simulink model "Simple_Model_Packaging_power_estimate"  (R2022b)
settings: Solver=VariableStepAuto  StartTime=0.0  StopTime=0.001  RelTol=1e-3
InitFcn:
  | Parameter_Initialize_1
undefined symbols (not defined in the file or in its folder): gcbh, magnitude, model, rcfiltgaincompat, rsgenpoly
libraries: simulink x5, commsynccomp2 x3, commblkcod2 x2, commfilt2 x2, commdigbbndam3 x2, commrandsrc3 x2, commseqgen3 x2, commsink2 x1, commdigbbndfm2 x1, commchan3 x1, dspsigops x1, commdigbbndcpm2 x1
settings Model: Creator=89778  LastModifiedBy=89778

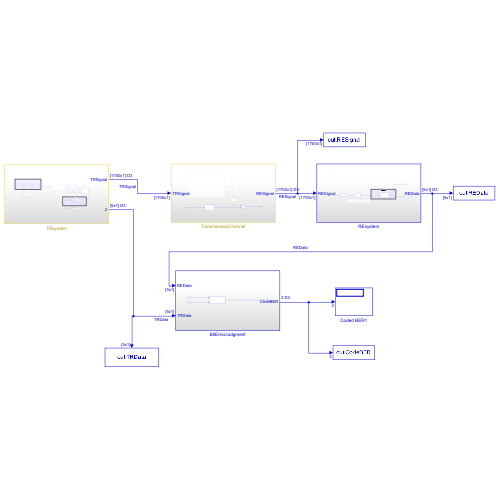
[thumbnail: Simulink's stored preview of the top-level diagram]
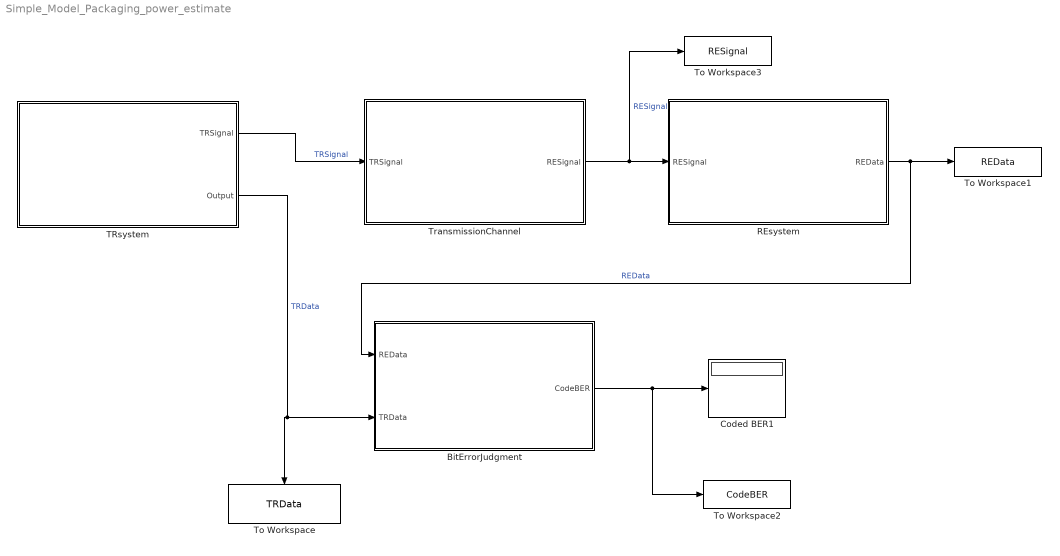
== system Simple_Model_Packaging_power_estimate ==
  BitErrorJudgment : Subsystem
  Coded BER1 : Display
  REsystem : Subsystem
  TRsystem : Subsystem
  To Workspace : ToWorkspace  VariableName=TRData  SaveFormat=Timeseries  SampleTime=-1
  To Workspace1 : ToWorkspace  VariableName=REData  SaveFormat=Timeseries  SampleTime=-1
  To Workspace2 : ToWorkspace  VariableName=CodeBER  SaveFormat=Timeseries  SampleTime=-1
  To Workspace3 : ToWorkspace  VariableName=RESignal  SaveFormat=Timeseries  SampleTime=-1
  TransmissionChannel : Subsystem
  wires:
  REsystem/1(REData) -> BitErrorJudgment/1(REData), To Workspace1/1  "REData"
  TransmissionChannel/1(RESignal) -> To Workspace3/1, REsystem/1(RESignal)  "RESignal"
  TRsystem/1(TRSignal) -> TransmissionChannel/1(TRSignal)  "TRSignal"
  TRsystem/2(Output) -> BitErrorJudgment/2(TRData), To Workspace/1  "TRData"
  BitErrorJudgment/1(CodeBER) -> To Workspace2/1, Coded BER1/1

== system Simple_Model_Packaging_power_estimate/BitErrorJudgment ==
  REData : Inport
  TRData : Inport  Port=2
  Bit Error Rate Calculation : Subsystem
      mask Display:
      | disp('Bit Error\nRate\nCalculation')
      | port_label('input', 1, 'Tx')
      | port_label('input', 2, 'Rx')
  CodeBER : Outport
  wires:
  TRData/1 -> Bit Error Rate Calculation/1(In1)
  REData/1 -> Bit Error Rate Calculation/2(In2)
  Bit Error Rate Calculation/1(Out1) -> CodeBER/1  "CodeBER"

== system Simple_Model_Packaging_power_estimate/REsystem ==
  note: 接收端解码
  note: 注意此处的延时设置，使得RS解码对齐信源部分，并在后续的码元比较时舍弃前三个编码周期(帧周期)的比特位
  RESignal : Inport
  Delay : Delay  DelayLength=model.Parameters.RE.Delay.Sample_length  InitialCondition=0  InputProcessing=Columns as channels (frame based)
  Integer-Output RS Decoder1 : commblkcod2/Integer-Output RS Decoder  n=model.Parameters.RE.Integer_Output_RS_Decoder1.Codeword_Length  k=model.Parameters.RE.Integer_Output_RS_Decoder1.Message_Length  specShortening=off  shortenedK=3  specGenPoly=off  genPoly=rsgenpoly(7, 3, [], [], 'double')  specPrimPoly=off  prPoly='X^3 + X + 1'  specPuncture=off  punctVec=[ones(2,1); zeros(2,1)]  specErasurePort=off  showNumErr=on
  Raised Cosine Receive Filter : commfilt2/Raised Cosine Receive Filter  filtType=Square root  R=model.Parameters.RE.Raised_Cosine_Receive_Filter.Rolloff_factor  filtSpan=model.Parameters.RE.Raised_Cosine_Receive_Filter.Filter_span_in_symbols  N=model.Parameters.RE.Raised_Cosine_Receive_Filter.Input_samples_per_symbol  downFactor=model.Parameters.RE.Raised_Cosine_Receive_Filter.Decimation_factor  downOffset=0  filterGain=rcfiltgaincompat(gcbh)  InputProcessing=Columns as channels (frame based)  RateOptions=Enforce single-rate processing  framing=Mute  checkCoeff=off  variableName=rcRxFilt  currentFiltSpan=10  D=5  inputOffset=0  sampMode=Mute  saveAsFlag=0  rateMode=Downsampling  checkGain=Normalized  launchFVT=on  roundingMode=Floor  overflowMode=off  coeffDataTypeStr=Inherit: Same word length as input  coeffMin=[]  coeffMax=[]  coeffLastDataTypeStr=Inherit: Same word length as input  accumDataTypeStr=Inherit: Same as product output  accumLastDataTypeStr=Inherit: Same as product output  outputDataTypeStr=Inherit: Same as accumulator  outputMin=[]  outputMax=[]  outputLastDataTypeStr=Inherit: Same as accumulator
  Rectangular QAM Demodulator Baseband : commdigbbndam3/Rectangular QAM Demodulator Baseband  M=model.Parameters.RE.Rectangular_QAM_Demodulator_Baseband.M_Number  OutType=Integer  DecType=Hard decision  VarSource=Dialog  Variance=1  Dec=Gray  Mapping=[0:15]  PowType=Min. distance between symbols  MinDist=model.Parameters.RE.Rectangular_QAM_Demodulator_Baseband.Minimum_distance  AvgPow=1  PeakPow=1  Ph=0  outDtype1=Inherit via internal rule  outDtype2=Inherit via internal rule  derotateFactorWordLen=16  derotateFactorDataTypeStr=Inherit: Same word length as input  derotateFactorLastDataTypeStr=Inherit: Same word length as input  denormFactorWordLen=16  denormFactorDataTypeStr=Inherit: Same word length as input  denormFactorLastDataTypeStr=Inherit: Same word length as input  prodOutWordLen=32  prodOutOverflowMode=Wrap  prodOutRoundingMode=Floor  prodOutOvFlMode=off  prodOutOvFlModeLastStrValue=off  sumWordLen=32
  Total Number of Corrected Errors : Display
  REData : Outport
  wires:
  Integer-Output RS Decoder1/2 -> Total Number of Corrected Errors/1
  Rectangular QAM Demodulator Baseband/1 -> Delay/1
  Delay/1 -> Integer-Output RS Decoder1/1
  Raised Cosine Receive Filter/1 -> Rectangular QAM Demodulator Baseband/1
  RESignal/1 -> Raised Cosine Receive Filter/1  "RESignal"
  Integer-Output RS Decoder1/1 -> REData/1  "REData"

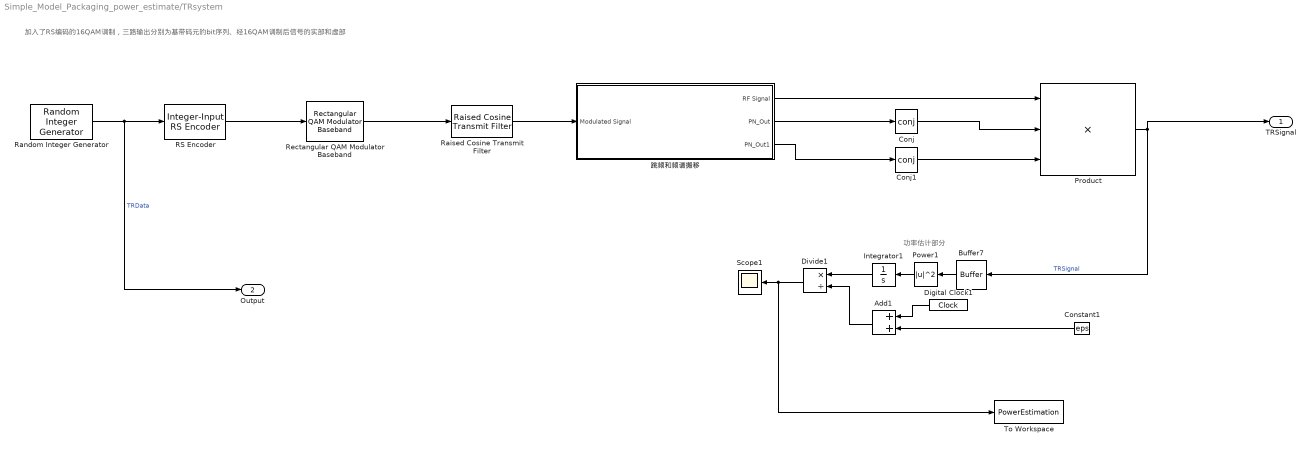
== system Simple_Model_Packaging_power_estimate/TRsystem ==
  note: 功率估计部分
  note: 加入了RS编码的16QAM调制，三路输出分别为基带码元的bit序列、经16QAM调制后信号的实部和虚部
  Add1 : Sum
  Buffer7 : Buffer  N=1  OutputFrames=off
  Conj : Math  Operator=conj
  Conj1 : Math  Operator=conj
  Constant1 : Constant  Value=eps  SampleTime=model.Parameters.TR.system_frame_speed
  Digital Clock1 : DigitalClock  SampleTime=model.Parameters.TR.system_frame_speed
  Divide1 : Product  Inputs=*/
  Integrator1 : Integrator
  Power1 : Math  Operator=magnitude^2
  Product : Product  Inputs=3
  RS Encoder : commblkcod2/Integer-Input RS Encoder  n=model.Parameters.TR.RS_Encoder.Codeword_Length  k=model.Parameters.TR.RS_Encoder.Message_Length  specShortening=off  shortenedK=3  specGenPoly=off  genPoly=rsgenpoly(7,3)  specPrimPoly=off  prPoly=[1 0 1 1]  specPuncture=off  punctVec=[ones(2,1); zeros(2,1)]
  Raised Cosine Transmit Filter : commfilt2/Raised Cosine Transmit Filter  filtType=Square root  R=model.Parameters.TR.Raised_Cosine_Transmit_Filter.Rolloff_factor  filtSpan=model.Parameters.TR.Raised_Cosine_Transmit_Filter.Filter_span_in_symbols  N=model.Parameters.TR.Raised_Cosine_Transmit_Filter.Output_samples_per_symbol  filterGain=rcfiltgaincompat(gcbh)  InputProcessing=Columns as channels (frame based)  RateOptions=Enforce single-rate processing  framing=Mute  checkCoeff=off  variableName=rcTxFilt  checkGain=Normalized  sampMode=Mute  saveAsFlag=0  currentFiltSpan=10  D=(10)/2  launchFVT=on  roundingMode=Floor  overflowMode=off  coeffDataTypeStr=Inherit: Same word length as input  coeffMin=[]  coeffMax=[]  coeffLastDataTypeStr=Inherit: Same word length as input  outputDataTypeStr=Inherit: Same as accumulator  outputMin=[]  outputMax=[]  outputLastDataTypeStr=Inherit: Same as accumulator
  Random Integer Generator : commrandsrc3/Random Integer Generator  SetSize=model.Parameters.TR.Random_Integer_Generator.SetSize  SeedSource=Auto  Seed=4  SampleTime=model.Parameters.TR.Random_Integer_Generator.Random_Sample_Time  SamplesPerFrame=model.Parameters.TR.Random_Integer_Generator.Samples_per_frame  OutputDataType=double  SimulateUsing=Interpreted execution
  Rectangular QAM Modulator Baseband : commdigbbndam3/Rectangular QAM Modulator Baseband  M=model.Parameters.TR.Rectangular_QAM_Modulator_Baseband.M_Number  InType=Integer  Enc=Gray  Mapping=[0:15]  PowType=Min. distance between symbols  MinDist=model.Parameters.TR.Rectangular_QAM_Modulator_Baseband.Minimum_distance  AvgPow=1  PeakPow=1  Ph=0  outDtype=double  outWordLen=16  outUDDataType=sfix(16)  outFracLenMode=Best precision  outFracLen=15  outDataTypeStr=double  outLastDataTypeStr=double
      settings: LibrarySourceBlock=|
      | commhdldigbbndam/Rectangular QAM
      | Modulator
      | Baseband
  Scope1 : Scope
  To Workspace : ToWorkspace  VariableName=PowerEstimation  SaveFormat=Timeseries  SampleTime=-1
  跳频和频谱搬移 : Subsystem
  TRSignal : Outport
  Output : Outport  Port=2
  wires:
  RS Encoder/1 -> Rectangular QAM Modulator Baseband/1
  跳频和频谱搬移/1(RF Signal) -> Product/1
  Random Integer Generator/1 -> Output/1, RS Encoder/1  "TRData"
  跳频和频谱搬移/3(PN_Out1) -> Conj1/1
  跳频和频谱搬移/2(PN_Out) -> Conj/1
  Raised Cosine Transmit Filter/1 -> 跳频和频谱搬移/1(Modulated Signal)
  Add1/1 -> Divide1/2
  Digital Clock1/1 -> Add1/1
  Divide1/1 -> To Workspace/1, Scope1/1
  Conj/1 -> Product/2
  Integrator1/1 -> Divide1/1
  Conj1/1 -> Product/3
  Constant1/1 -> Add1/2
  Rectangular QAM Modulator Baseband/1 -> Raised Cosine Transmit Filter/1
  Product/1 -> TRSignal/1, Buffer7/1  "TRSignal"
  Buffer7/1 -> Power1/1
  Power1/1 -> Integrator1/1

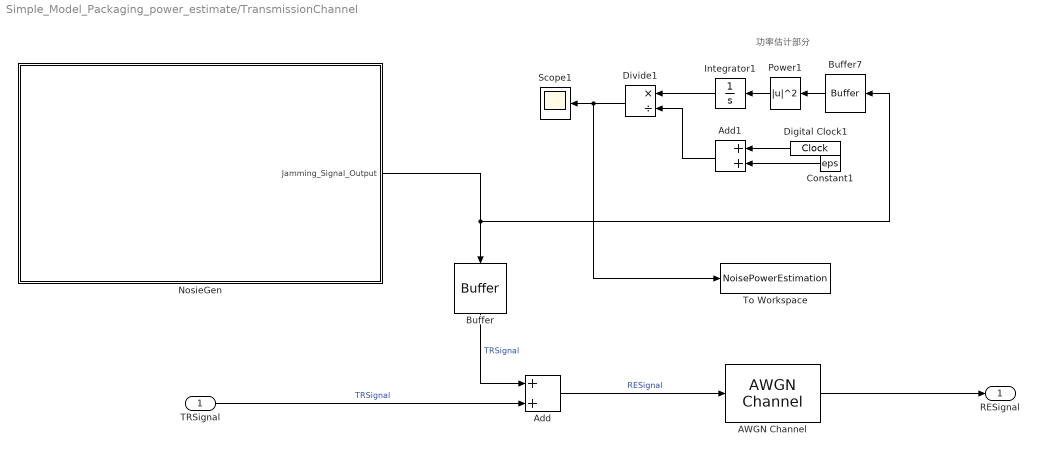
== system Simple_Model_Packaging_power_estimate/TransmissionChannel ==
  note: 功率估计部分
  TRSignal : Inport
  AWGN Channel : commchan3/AWGN Channel  InputProcessing=Columns as channels (frame based)  seed=67  noiseMode="Signal to noise ratio  (SNR)"  EbNodB=10  EsNodB=10  SNRdB=model.Parameters.Channel.Awgn.SNR  bitsPerSym=1  Ps=model.Parameters.Channel.Awgn.input_power  Tsym=1  variance=1
  Add : Sum
  Add1 : Sum
  Buffer : Buffer  N=model.Parameters.TR.rolloff_later_data_length  OutputFrames=off
  Buffer7 : Buffer  N=1  OutputFrames=off
  Constant1 : Constant  Value=eps  SampleTime=model.Parameters.TR.system_frame_speed
  Digital Clock1 : DigitalClock  SampleTime=model.Parameters.NoiseGen.NoiseTs
  Divide1 : Product  Inputs=*/
  Integrator1 : Integrator
  NosieGen : Subsystem
  Power1 : Math  Operator=magnitude^2
  Scope1 : Scope
  To Workspace : ToWorkspace  VariableName=NoisePowerEstimation  SaveFormat=Timeseries  SampleTime=-1
  RESignal : Outport
  wires:
  Add/1 -> AWGN Channel/1  "RESignal"
  NosieGen/1(Jamming_Signal_Output) -> Buffer7/1, Buffer/1
  AWGN Channel/1 -> RESignal/1
  TRSignal/1 -> Add/2  "TRSignal"
  Buffer/1 -> Add/1  "TRSignal"
  Power1/1 -> Integrator1/1
  Add1/1 -> Divide1/2
  Buffer7/1 -> Power1/1
  Divide1/1 -> To Workspace/1, Scope1/1
  Constant1/1 -> Add1/2
  Integrator1/1 -> Divide1/1
  Digital Clock1/1 -> Add1/1

== system Simple_Model_Packaging_power_estimate/BitErrorJudgment/Bit Error Rate Calculation ==
  In1 : Inport
  In2 : Inport  Port=2
  Error Rate Calculation : commsink2/Error Rate Calculation  N=model.Parameters.BER.Error_Rate_Calculation.receive_Delay  st_delay=0  cp_mode=Entire frame  subframe=[]  PMode=Port  WsName=ErrorVec  RsMode2=off  stop=on  numErr=100  maxBits=1e9
  Integer to Bit Converter : simulink/Logic and Bit Operations/Integer to Bit Converter  nbits=model.Parameters.BER.Integer_to_Bit_Converter.M  signedInputValues=Unsigned  bitOrder=MSB first  outDtype=Inherit via internal rule
      settings: LibrarySourceBlock=|
      | commutil2/Integer to Bit
      | Converter
  Integer to Bit Converter1 : simulink/Logic and Bit Operations/Integer to Bit Converter  nbits=model.Parameters.BER.Integer_to_Bit_Converter1.M  signedInputValues=Unsigned  bitOrder=MSB first  outDtype=Inherit via internal rule
      settings: LibrarySourceBlock=|
      | commutil2/Integer to Bit
      | Converter
  Out1 : Outport  VectorParamsAs1DForOutWhenUnconnected=off
  wires:
  Integer to Bit Converter/1 -> Error Rate Calculation/1
  Integer to Bit Converter1/1 -> Error Rate Calculation/2
  In1/1 -> Integer to Bit Converter/1
  Error Rate Calculation/1 -> Out1/1
  In2/1 -> Integer to Bit Converter1/1

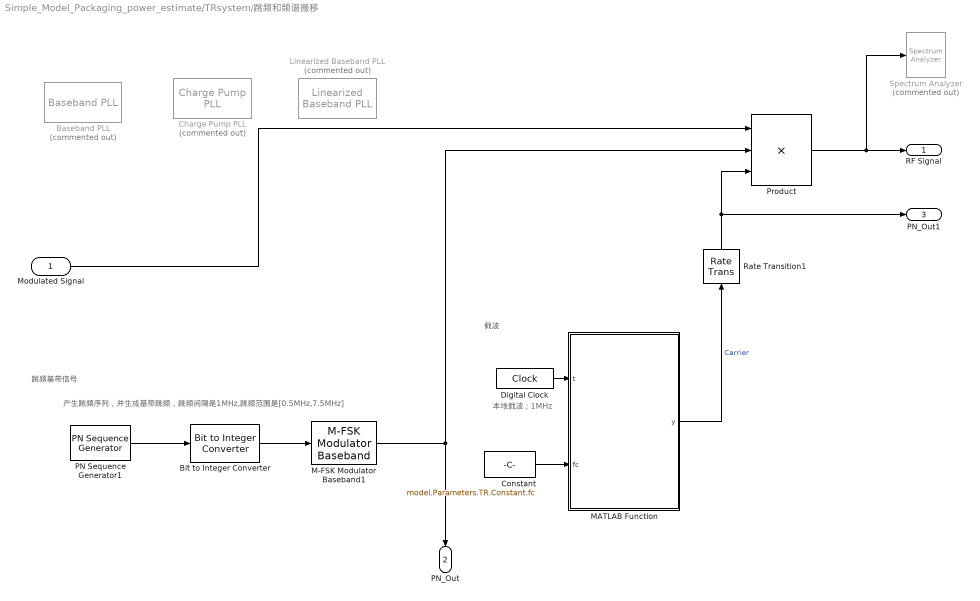
== system Simple_Model_Packaging_power_estimate/TRsystem/跳频和频谱搬移 ==
  note: 本地载波 ; 1MHz
  note: 产生跳频序列，并生成基带跳频，跳频间隔是1MHz,跳频范围是[0.5MHz,7.5MHz]
  note: 跳频基带信号
  note: 载波
  Modulated Signal : Inport
  Baseband PLL : commsynccomp2/Baseband PLL  Commented=on  Fn="[3.0002  0  40002]"  Fd="[1   67.46   2270.9   40002]"  Kvco=1
  Bit to Integer Converter : simulink/Logic and Bit Operations/Bit to Integer Converter  nbits=model.Parameters.TR.Bit_to_Integer_Converter.M  bitOrder=MSB first  signedOutputValues=Unsigned  outDtype=double  outDtypeSigned=Inherit via internal rule
  Charge Pump PLL : commsynccomp2/Charge Pump PLL  Commented=on  Fn="[3.0002  0  40002]"  Fd="[1   67.46   2270.9   40002]"  Kvco=1  Fc=100  Ph=0  Ac=1
  Constant : Constant  Value=model.Parameters.TR.Constant.fc
  Digital Clock : DigitalClock  SampleTime=model.Parameters.TR.Digital_Clock.fc_Ts
  Linearized Baseband PLL : commsynccomp2/Linearized Baseband PLL  Commented=on  Fn="[3.0002  0  40002]"  Fd="[1   67.46   2270.9   40002]"  Kvco=1
  M-FSK Modulator Baseband1 : commdigbbndfm2/M-FSK Modulator Baseband  M=model.Parameters.TR.M_FSK_Modulator_Baseband1.M_ary_number  InType=Integer  Enc=Gray  freqSep=model.Parameters.TR.M_FSK_Modulator_Baseband1.Frequency_separation  phaseType=Continuous  numSamp=model.Parameters.TR.M_FSK_Modulator_Baseband1.Samples_per_symbol  RateOptions=Enforce single-rate processing  outDataType=double
  MATLAB Function : MATLAB Function  TreatAsAtomicUnit=on
  PN Sequence Generator1 : commseqgen3/PN Sequence Generator  poly=model.Parameters.TR.PN_Sequence_Generator1.Generator_polynomial  ini_sta=model.Parameters.TR.PN_Sequence_Generator1.Initial_states  outBitMaskSource=Dialog parameter  shift=0  outVarSiz=off  maxOutSizeMode=Dialog parameter  maxOutSize=[10 1]  Ts=model.Parameters.TR.PN_Sequence_Generator1.Sample_time  sampPerFrame=model.Parameters.TR.PN_Sequence_Generator1.Samples_per_frame  reset=off  bitPackedOutputs=off  outDataType=double  numPackedBits=5  bitPackDataSigned=off  bitPackedOutDType=double
  Product : Product  Inputs=3
  Rate Transition1 : RateTransition
  Spectrum Analyzer : SpectrumAnalyzer  Commented=on
  RF Signal : Outport
  PN_Out : Outport  Port=2
  PN_Out1 : Outport  Port=3
  wires:
  Bit to Integer Converter/1 -> M-FSK Modulator Baseband1/1
  PN Sequence Generator1/1 -> Bit to Integer Converter/1
  Modulated Signal/1 -> Product/1
  Product/1 -> Spectrum Analyzer/1, RF Signal/1
  Digital Clock/1 -> MATLAB Function/1(t)
  M-FSK Modulator Baseband1/1 -> Product/2, PN_Out/1
  MATLAB Function/1(y) -> Rate Transition1/1  "Carrier"
  Rate Transition1/1 -> Product/3, PN_Out1/1
  Constant/1 -> MATLAB Function/2(fc)

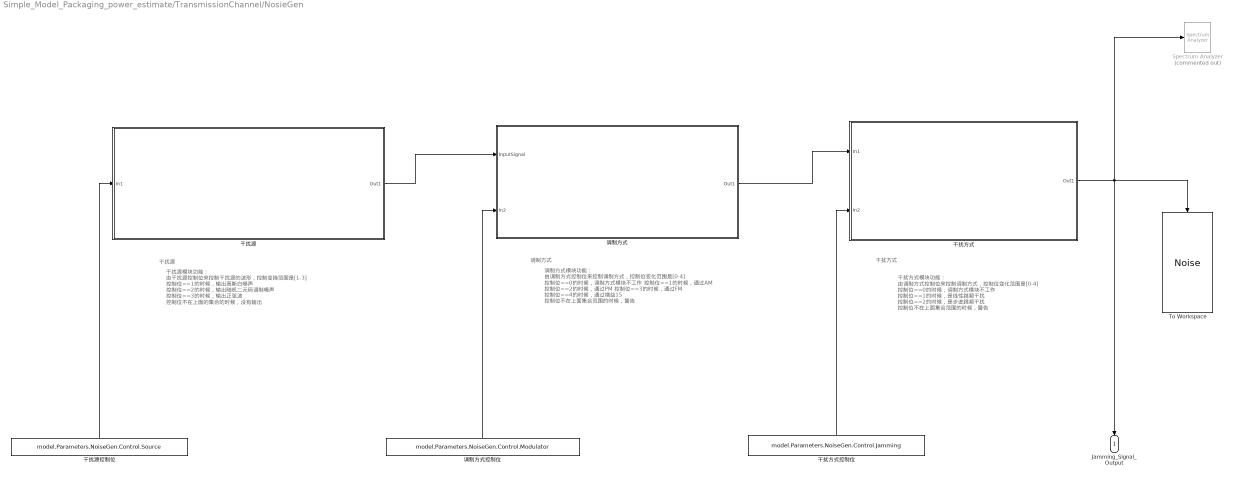
== system Simple_Model_Packaging_power_estimate/TransmissionChannel/NosieGen ==
  note: 干扰方式模块功能：
      | 由调制方式控制位来控制调制方式，控制位变化范围是[0-4]
      | 控制位==0的时候，调制方式模块不工作
      | 控制位==1的时候，是线性跳频干扰
      | 控制位==2的时候，是步进跳频干扰
      | 控制位不在上面集合范围的时候，警告
  note: 干扰源模块功能：
      | 由干扰源控制位来控制干扰源的波形，控制变换范围是[1-3]
      | 控制位==1的时候，输出高斯白噪声
      | 控制位==2的时候，输出随机二元码调制噪声
      | 控制位==3的时候，输出正弦波
      | 控制位不在上面的集合的时候，没有输出
  note: 调制方式模块功能：
      | 由调制方式控制位来控制调制方式，控制位变化范围是[0-4]
      | 控制位==0的时候，调制方式模块不工作
      | 控制位==1的时候，通过AM
      | 控制位==2的时候，通过PM
      | 控制位==3的时候，通过FM
      | 控制位==4的时候，通过增益15
      | 控制位不在上面集合范围的时候，警告
  note: 干扰方式
  note: 干扰源
  note: 调制方式
  Spectrum Analyzer : SpectrumAnalyzer  Commented=on
  To Workspace : ToWorkspace  VariableName=Noise  SaveFormat=Timeseries  SampleTime=-1
  干扰方式 : Subsystem
  干扰方式控制位 : Constant  Value=model.Parameters.NoiseGen.Control.Jamming  SampleTime=Inf
  干扰源 : Subsystem
  干扰源控制位 : Constant  Value=model.Parameters.NoiseGen.Control.Source  SampleTime=Inf
  调制方式 : Subsystem
  调制方式控制位 : Constant  Value=model.Parameters.NoiseGen.Control.Modulator  SampleTime=Inf
  Jamming_Signal_Output : Outport
  wires:
  干扰方式/1(Out1) -> To Workspace/1, Jamming_Signal_Output/1, Spectrum Analyzer/1
  调制方式/1(Out1) -> 干扰方式/1(In1)
  干扰源/1(Out1) -> 调制方式/1(InputSignal)
  干扰方式控制位/1 -> 干扰方式/2(In2)
  干扰源控制位/1 -> 干扰源/1(In1)
  调制方式控制位/1 -> 调制方式/2(In2)

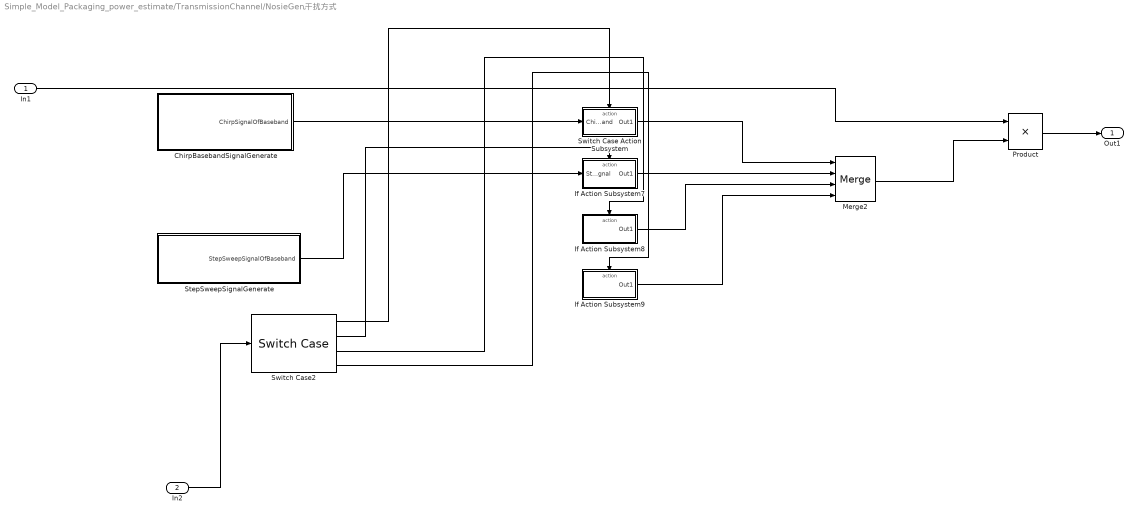
== system Simple_Model_Packaging_power_estimate/TransmissionChannel/NosieGen/干扰方式 ==
  In1 : Inport
  In2 : Inport  Port=2
  ChirpBasebandSignalGenerate : Subsystem
      settings: AttributesFormatString=|
      | 线性调频模块：线性调频公式(y=exp(2*pi*(f_min*t+0.5*k_chirp*t^2)))
      | 输入参数：
      | 1. f_min,为线性调频信号的起始频率
      | 2.f_max为线性调频信号的终止频率
      | 3.T_chirp为线性调频信号的调频时间
      | 斜率k_sweep = (f_min-f_max)/T_chirp
  If Action Subsystem7 : Subsystem  TreatAsAtomicUnit=on
  If Action Subsystem8 : Subsystem  TreatAsAtomicUnit=on
  If Action Subsystem9 : Subsystem  TreatAsAtomicUnit=on
  Merge2 : Merge  Inputs=4
  Product : Product
  StepSweepSignalGenerate : Subsystem
  Switch Case Action Subsystem : Subsystem  TreatAsAtomicUnit=on
  Switch Case2 : SwitchCase  CaseConditions={1,2,3}
  Out1 : Outport
  wires:
  If Action Subsystem9/1(Out1) -> Merge2/4
  Switch Case Action Subsystem/1(Out1) -> Merge2/1
  If Action Subsystem8/1(Out1) -> Merge2/3
  Switch Case2/3 -> If Action Subsystem8/Action
  Switch Case2/1 -> Switch Case Action Subsystem/Action
  Switch Case2/2 -> If Action Subsystem7/Action
  Switch Case2/4 -> If Action Subsystem9/Action
  ChirpBasebandSignalGenerate/1(ChirpSignalOfBaseband) -> Switch Case Action Subsystem/1(ChirpSignalOfBaseband)
  If Action Subsystem7/1(Out1) -> Merge2/2
  Merge2/1 -> Product/2
  Product/1 -> Out1/1
  In1/1 -> Product/1
  In2/1 -> Switch Case2/1
  StepSweepSignalGenerate/1(StepSweepSignalOfBaseband) -> If Action Subsystem7/1(StepSweepSignal)

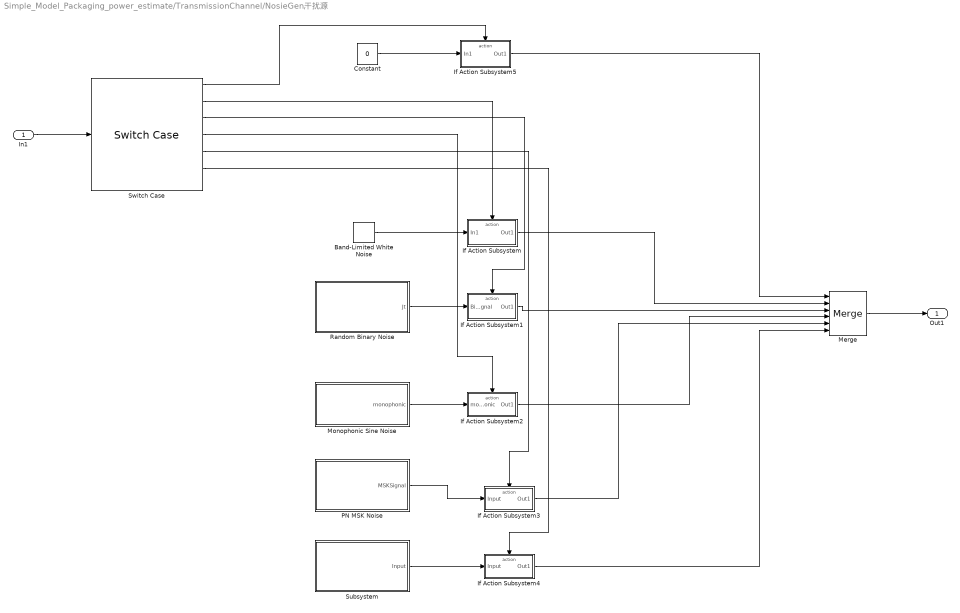
== system Simple_Model_Packaging_power_estimate/TransmissionChannel/NosieGen/干扰源 ==
  In1 : Inport
  Band-Limited White Noise : simulink/Sources/Band-Limited White Noise  Cov=model.Parameters.NoiseGen.GaussPower  Ts=model.Parameters.NoiseGen.NoiseTs  seed=model.Parameters.NoiseGen.GaussSeed
  Constant : Constant  Value=0  SampleTime=model.Parameters.NoiseGen.NoiseTs
  If Action Subsystem : Subsystem  TreatAsAtomicUnit=on
  If Action Subsystem1 : Subsystem  TreatAsAtomicUnit=on
  If Action Subsystem2 : Subsystem  TreatAsAtomicUnit=on
  If Action Subsystem3 : Subsystem  TreatAsAtomicUnit=on
  If Action Subsystem4 : Subsystem  TreatAsAtomicUnit=on
  If Action Subsystem5 : Subsystem  TreatAsAtomicUnit=on
  Merge : Merge  Inputs=6
  Monophonic Sine Noise : Subsystem
  PN MSK Noise : Subsystem
  Random Binary Noise : Subsystem
  Subsystem : Subsystem
  Switch Case : SwitchCase  CaseConditions={0,1,2,3,4,5}
  Out1 : Outport
  wires:
  Switch Case/3 -> If Action Subsystem1/Action
  If Action Subsystem2/1(Out1) -> Merge/4
  Band-Limited White Noise/1 -> If Action Subsystem/1(In1)
  If Action Subsystem1/1(Out1) -> Merge/3
  Random Binary Noise/1(Jt) -> If Action Subsystem1/1(Binary_Random_Signal)
  Switch Case/4 -> If Action Subsystem2/Action
  Switch Case/2 -> If Action Subsystem/Action
  Merge/1 -> Out1/1
  In1/1 -> Switch Case/1
  Monophonic Sine Noise/1(monophonic) -> If Action Subsystem2/1(monophonic)
  Switch Case/5 -> If Action Subsystem3/Action
  If Action Subsystem3/1(Out1) -> Merge/5
  If Action Subsystem/1(Out1) -> Merge/2
  PN MSK Noise/1(MSKSignal) -> If Action Subsystem3/1(Input)
  Switch Case/6 -> If Action Subsystem4/Action
  Subsystem/1(Input) -> If Action Subsystem4/1(Input)
  If Action Subsystem4/1(Out1) -> Merge/6
  Switch Case/1 -> If Action Subsystem5/Action
  Constant/1 -> If Action Subsystem5/1(In1)
  If Action Subsystem5/1(Out1) -> Merge/1

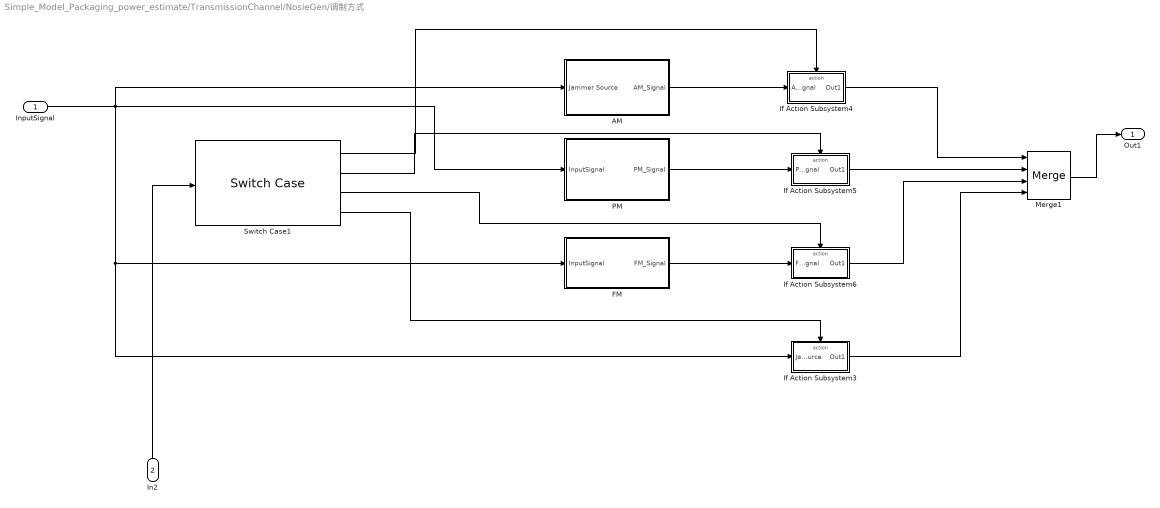
== system Simple_Model_Packaging_power_estimate/TransmissionChannel/NosieGen/调制方式 ==
  InputSignal : Inport
  In2 : Inport  Port=2
  AM : Subsystem
  FM : Subsystem
  If Action Subsystem3 : Subsystem  TreatAsAtomicUnit=on
  If Action Subsystem4 : Subsystem  TreatAsAtomicUnit=on
  If Action Subsystem5 : Subsystem  TreatAsAtomicUnit=on
  If Action Subsystem6 : Subsystem  TreatAsAtomicUnit=on
  Merge1 : Merge  Inputs=4
  PM : Subsystem
  Switch Case1 : SwitchCase  CaseConditions={1,2,3}
  Out1 : Outport
  wires:
  In2/1 -> Switch Case1/1
  PM/1(PM_Signal) -> If Action Subsystem5/1(PM_Signal)
  Merge1/1 -> Out1/1
  If Action Subsystem3/1(Out1) -> Merge1/4
  If Action Subsystem6/1(Out1) -> Merge1/3
  If Action Subsystem5/1(Out1) -> Merge1/2
  InputSignal/1 -> FM/1(InputSignal), If Action Subsystem3/1(Jammer Source), PM/1(InputSignal), AM/1(Jammer Source)
  AM/1(AM_Signal) -> If Action Subsystem4/1(AM_Signal)
  Switch Case1/2 -> If Action Subsystem5/Action
  Switch Case1/3 -> If Action Subsystem6/Action
  Switch Case1/1 -> If Action Subsystem4/Action
  If Action Subsystem4/1(Out1) -> Merge1/1
  FM/1(FM_Signal) -> If Action Subsystem6/1(FM_Signal)
  Switch Case1/4 -> If Action Subsystem3/Action

== system Simple_Model_Packaging_power_estimate/TransmissionChannel/NosieGen/干扰方式/ChirpBasebandSignalGenerate ==
  note: 线性调频模块：线性调频公式(y=exp(2*pi*(fmin*t+0.5*k_chirp*t^2)))
      | 输入参数：
      | 1.fmin,为线性调频信号的起始频率
      | 2.fmax为线性调频信号的终止频率
      | 3.T_chirp为线性调频信号的调频时间
      | 斜率k_sweep = (f_min-f_max)/T_chirp
  note: 线性调频模块
  Chirp_Signal_Generation : MATLAB Function  TreatAsAtomicUnit=on
  Constant : Constant  Value=model.Parameters.NoiseGen.Jamming.LinearSweepFmin
  Constant1 : Constant  Value=model.Parameters.NoiseGen.Jamming.LinearSweepT
  Constant2 : Constant  Value=model.Parameters.NoiseGen.Jamming.LinearSweepK
  Digital Clock : DigitalClock  SampleTime=model.Parameters.NoiseGen.NoiseTs
  Frequency_Check : Subsystem  Commented=on
  ChirpSignalOfBaseband : Outport
  wires:
  Digital Clock/1 -> Chirp_Signal_Generation/1(t)
  Chirp_Signal_Generation/1(y) -> ChirpSignalOfBaseband/1  "ChirpSignal"
  Frequency_Check/1(FrequencyConversionLine) -> ?
  Constant/1 -> Chirp_Signal_Generation/2(f_chirp_min)
  Constant2/1 -> Chirp_Signal_Generation/4(k_chirp)
  Constant1/1 -> Chirp_Signal_Generation/3(T_chirp)

== system Simple_Model_Packaging_power_estimate/TransmissionChannel/NosieGen/干扰方式/If Action Subsystem7 ==
  StepSweepSignal : Inport
  Action Port : ActionPort  ActionPortLabel=case [ 2 ]:
  Out1 : Outport
  wires:
  StepSweepSignal/1 -> Out1/1

== system Simple_Model_Packaging_power_estimate/TransmissionChannel/NosieGen/干扰方式/If Action Subsystem8 ==
  Action Port : ActionPort  ActionPortLabel=case [ 3 ]:
  Constant : Constant  Value=10
  Constant1 : Constant  Value=0
  Real-Imag to Complex : RealImagToComplex
  Out1 : Outport
  wires:
  Constant/1 -> Real-Imag to Complex/1
  Real-Imag to Complex/1 -> Out1/1
  Constant1/1 -> Real-Imag to Complex/2

== system Simple_Model_Packaging_power_estimate/TransmissionChannel/NosieGen/干扰方式/If Action Subsystem9 ==
  Action Port : ActionPort  ActionPortLabel=default:
  Constant : Constant
  Constant1 : Constant  Value=0
  Real-Imag to Complex : RealImagToComplex
  Out1 : Outport
  wires:
  Constant/1 -> Real-Imag to Complex/1
  Real-Imag to Complex/1 -> Out1/1
  Constant1/1 -> Real-Imag to Complex/2

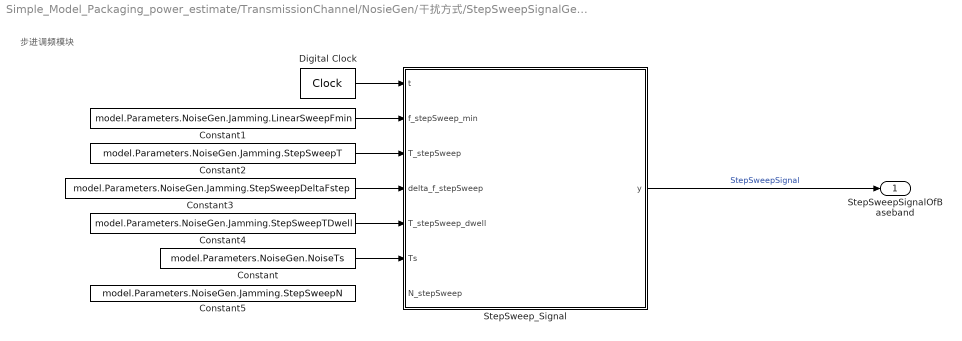
== system Simple_Model_Packaging_power_estimate/TransmissionChannel/NosieGen/干扰方式/StepSweepSignalGenerate ==
  note: 步进调频模块
  Constant : Constant  Value=model.Parameters.NoiseGen.NoiseTs
  Constant1 : Constant  Value=model.Parameters.NoiseGen.Jamming.LinearSweepFmin
  Constant2 : Constant  Value=model.Parameters.NoiseGen.Jamming.StepSweepT
  Constant3 : Constant  Value=model.Parameters.NoiseGen.Jamming.StepSweepDeltaFstep
  Constant4 : Constant  Value=model.Parameters.NoiseGen.Jamming.StepSweepTDwell
  Constant5 : Constant  Value=model.Parameters.NoiseGen.Jamming.StepSweepN
  Digital Clock : DigitalClock  SampleTime=model.Parameters.NoiseGen.NoiseTs
  StepSweep_Signal : MATLAB Function  TreatAsAtomicUnit=on
  StepSweepSignalOfBaseband : Outport
  wires:
  Digital Clock/1 -> StepSweep_Signal/1(t)
  StepSweep_Signal/1(y) -> StepSweepSignalOfBaseband/1  "StepSweepSignal"
  Constant/1 -> StepSweep_Signal/6(Ts)
  Constant1/1 -> StepSweep_Signal/2(f_stepSweep_min)
  Constant2/1 -> StepSweep_Signal/3(T_stepSweep)
  Constant3/1 -> StepSweep_Signal/4(delta_f_stepSweep)
  Constant4/1 -> StepSweep_Signal/5(T_stepSweep_dwell)

== system Simple_Model_Packaging_power_estimate/TransmissionChannel/NosieGen/干扰方式/Switch Case Action Subsystem ==
  ChirpSignalOfBaseband : Inport
  Action Port : ActionPort  ActionPortLabel=case [ 1 ]:
  Out1 : Outport
  wires:
  ChirpSignalOfBaseband/1 -> Out1/1

== system Simple_Model_Packaging_power_estimate/TransmissionChannel/NosieGen/干扰源/If Action Subsystem ==
  In1 : Inport
  Action Port : ActionPort  ActionPortLabel=case [ 1 ]:
  Out1 : Outport
  wires:
  In1/1 -> Out1/1

== system Simple_Model_Packaging_power_estimate/TransmissionChannel/NosieGen/干扰源/If Action Subsystem1 ==
  Binary_Random_Signal : Inport
  Action Port : ActionPort  ActionPortLabel=case [ 2 ]:
  Out1 : Outport
  wires:
  Binary_Random_Signal/1 -> Out1/1

== system Simple_Model_Packaging_power_estimate/TransmissionChannel/NosieGen/干扰源/If Action Subsystem2 ==
  monophonic : Inport
  Action Port : ActionPort  ActionPortLabel=case [ 3 ]:
  Out1 : Outport
  wires:
  monophonic/1 -> Out1/1

== system Simple_Model_Packaging_power_estimate/TransmissionChannel/NosieGen/干扰源/If Action Subsystem3 ==
  Input : Inport
  Action Port : ActionPort  ActionPortLabel=case [ 4 ]:
  Out1 : Outport
  wires:
  Input/1 -> Out1/1

== system Simple_Model_Packaging_power_estimate/TransmissionChannel/NosieGen/干扰源/If Action Subsystem4 ==
  Input : Inport
  Action Port : ActionPort  ActionPortLabel=case [ 5 ]:
  Out1 : Outport
  wires:
  Input/1 -> Out1/1

== system Simple_Model_Packaging_power_estimate/TransmissionChannel/NosieGen/干扰源/If Action Subsystem5 ==
  In1 : Inport
  Action Port : ActionPort  ActionPortLabel=case [ 0 ]:
  Out1 : Outport
  wires:
  In1/1 -> Out1/1

== system Simple_Model_Packaging_power_estimate/TransmissionChannel/NosieGen/干扰源/Monophonic Sine Noise ==
  Constant : Constant  Value=model.Parameters.NoiseGen.SineNoisePhi0
  Constant1 : Constant  Value=model.Parameters.NoiseGen.SineNoiseF
  Constant2 : Constant  Value=model.Parameters.NoiseGen.SineNoiseA
  Digital Clock : DigitalClock  SampleTime=model.Parameters.NoiseGen.NoiseTs
  Monophonic_Generate : MATLAB Function  TreatAsAtomicUnit=on
  monophonic : Outport
  wires:
  Digital Clock/1 -> Monophonic_Generate/1(t)
  Constant/1 -> Monophonic_Generate/4(phi0)
  Constant2/1 -> Monophonic_Generate/2(A)
  Constant1/1 -> Monophonic_Generate/3(freq)
  Monophonic_Generate/1(monophonic) -> monophonic/1

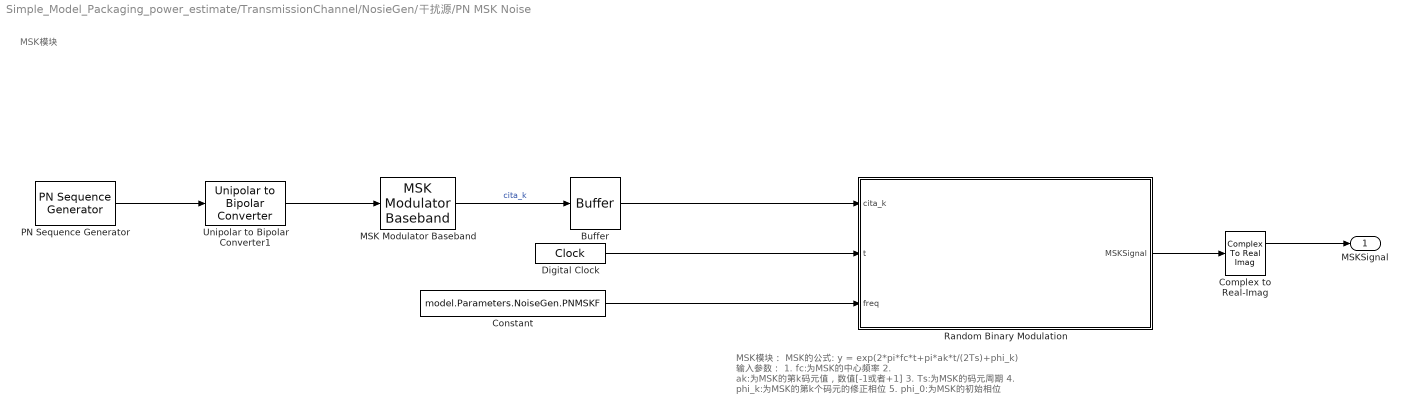
== system Simple_Model_Packaging_power_estimate/TransmissionChannel/NosieGen/干扰源/PN MSK Noise ==
  note: MSK模块
  note: MSK模块：
      | MSK的公式: y = exp(2*pi*fc*t+pi*ak*t/(2Ts)+phi_k)
      | 输入参数：
      | 1. fc:为MSK的中心频率
      | 2. ak:为MSK的第k码元值，数值[-1或者+1]
      | 3. Ts:为MSK的码元周期
      | 4. phi_k:为MSK的第k个码元的修正相位
      | 5. phi_0:为MSK的初始相位
  Buffer : Buffer  N=1  OutputFrames=off
  Complex to Real-Imag : ComplexToRealImag
  Constant : Constant  Value=model.Parameters.NoiseGen.PNMSKF
  Digital Clock : DigitalClock  SampleTime=model.Parameters.NoiseGen.NoiseTs
  MSK Modulator Baseband : commdigbbndcpm2/MSK Modulator Baseband  inputType=Integer  phaseOffset=model.Parameters.NoiseGen.PNMSKPhi0  samplesPerSymbol=model.Parameters.NoiseGen.PNMSKM  RateOptions=Enforce single-rate processing  outDataType=double
  PN Sequence Generator : commseqgen3/PN Sequence Generator  poly=model.Parameters.NoiseGen.PNMSKPolynomial  ini_sta=model.Parameters.NoiseGen.PNMSKInitialstate  outBitMaskSource=Dialog parameter  shift=0  outVarSiz=off  maxOutSizeMode=Dialog parameter  maxOutSize=[10 1]  Ts=model.Parameters.NoiseGen.PNMSKM * model.Parameters.NoiseGen.NoiseTs  sampPerFrame=1  reset=off  bitPackedOutputs=off  outDataType=double  numPackedBits=8  bitPackDataSigned=off  bitPackedOutDType=double
      settings: LibrarySourceBlock=|
      | commhdlsource/PN Sequence
      | Generator
  Random Binary Modulation : MATLAB Function  TreatAsAtomicUnit=on
  Unipolar to Bipolar Converter1 : commutil2/Unipolar to Bipolar Converter  M=2  polarity=Positive  dataType=Inherit via internal rule
  MSKSignal : Outport  OutDataTypeStr=double
  wires:
  Digital Clock/1 -> Random Binary Modulation/2(t)
  Unipolar to Bipolar Converter1/1 -> MSK Modulator Baseband/1
  PN Sequence Generator/1 -> Unipolar to Bipolar Converter1/1
  Constant/1 -> Random Binary Modulation/3(freq)
  MSK Modulator Baseband/1 -> Buffer/1  "cita_k"
  Buffer/1 -> Random Binary Modulation/1(cita_k)
  Random Binary Modulation/1(MSKSignal) -> Complex to Real-Imag/1
  Complex to Real-Imag/1 -> MSKSignal/1

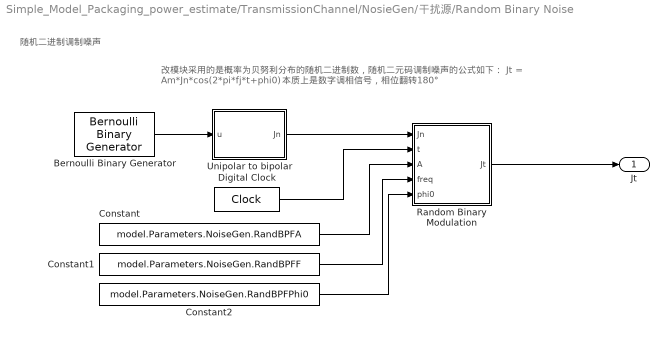
== system Simple_Model_Packaging_power_estimate/TransmissionChannel/NosieGen/干扰源/Random Binary Noise ==
  note: 改模块采用的是概率为贝努利分布的随机二进制数，随机二元码调制噪声的公式如下：
      | Jt = Am*Jn*cos(2*pi*fj*t+phi0)
      | 本质上是数字调相信号，相位翻转180°
  note: 随机二进制调制噪声
  Bernoulli Binary Generator : commrandsrc3/Bernoulli Binary Generator  ProbabilityOfZero=0.5  SeedSource=Auto  Seed=0  SampleTime=model.Parameters.NoiseGen.NoiseTs  SamplesPerFrame=1  OutputDataType=double  SimulateUsing=Interpreted execution
  Constant : Constant  Value=model.Parameters.NoiseGen.RandBPFA
  Constant1 : Constant  Value=model.Parameters.NoiseGen.RandBPFF
  Constant2 : Constant  Value=model.Parameters.NoiseGen.RandBPFPhi0
  Digital Clock : DigitalClock  SampleTime=model.Parameters.NoiseGen.NoiseTs
  Random Binary Modulation : MATLAB Function  TreatAsAtomicUnit=on
  Unipolar to bipolar : MATLAB Function  TreatAsAtomicUnit=on
  Jt : Outport
  wires:
  Unipolar to bipolar/1(Jn) -> Random Binary Modulation/1(Jn)
  Bernoulli Binary Generator/1 -> Unipolar to bipolar/1(u)
  Random Binary Modulation/1(Jt) -> Jt/1
  Digital Clock/1 -> Random Binary Modulation/2(t)
  Constant/1 -> Random Binary Modulation/3(A)
  Constant1/1 -> Random Binary Modulation/4(freq)
  Constant2/1 -> Random Binary Modulation/5(phi0)

== system Simple_Model_Packaging_power_estimate/TransmissionChannel/NosieGen/干扰源/Subsystem ==
  Band-Limited White Noise : simulink/Sources/Band-Limited White Noise  Cov=model.Parameters.NoiseGen.RFNoisePower  Ts=model.Parameters.NoiseGen.NoiseTs  seed=model.Parameters.NoiseGen.RFNoiseSeed
  Filter : dsparch4/Biquad Filter  Tag=BlockMethodSubSystem  FilterSource=Filter object  CoeffSource=Specify via dialog  FilterObject=model.Parameters.NoiseGen.RFNoiseFilterObj  IIRFiltStruct=Direct form II  BiQuadCoeffs=[1 2 1 1 -1.48178412853867569 0.831585910854089061;1 2 1 1 -1.27721148327892942 0.578720214976092495;1 2 1 1 -1.14298050253990113 0.412801598096188771;1 2 1 1 -1.06189684687510177 0.31257668783031084;1 2 1 1 -1.02371666858405952 0.265383392069520774]  ScaleValues=[0.0874504455788533558;0.0753771829242907976;0.0674552738890718956;0.0626699602388022664;0.0604166808713653344;1]  IC=0  ICnum=0  ICden=0  a0Flag=Warning  optimizeScaleValues=on  ScaleValueMode=Specify via input port (g)  roundingMode=Floor  overflowMode=off  scaleValueFracLength=14  denProdOutputFracLength=30  denAccumFracLength=30  secondMemoryFracLength=15
  Input : Outport
  wires:
  Band-Limited White Noise/1 -> Filter/1
  Filter/1 -> Input/1

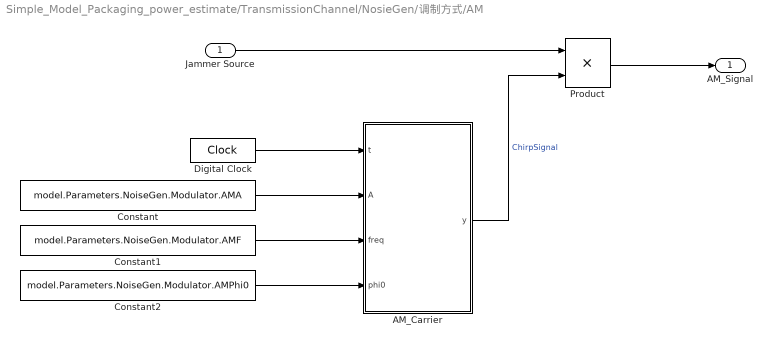
== system Simple_Model_Packaging_power_estimate/TransmissionChannel/NosieGen/调制方式/AM ==
  Jammer Source : Inport
  AM_Carrier : MATLAB Function  TreatAsAtomicUnit=on
  Constant : Constant  Value=model.Parameters.NoiseGen.Modulator.AMA
  Constant1 : Constant  Value=model.Parameters.NoiseGen.Modulator.AMF
  Constant2 : Constant  Value=model.Parameters.NoiseGen.Modulator.AMPhi0
  Digital Clock : DigitalClock  SampleTime=model.Parameters.NoiseGen.NoiseTs
  Product : Product
  AM_Signal : Outport
  wires:
  Digital Clock/1 -> AM_Carrier/1(t)
  AM_Carrier/1(y) -> Product/2  "ChirpSignal"
  Jammer Source/1 -> Product/1
  Product/1 -> AM_Signal/1
  Constant2/1 -> AM_Carrier/4(phi0)
  Constant1/1 -> AM_Carrier/3(freq)
  Constant/1 -> AM_Carrier/2(A)

== system Simple_Model_Packaging_power_estimate/TransmissionChannel/NosieGen/调制方式/FM ==
  InputSignal : Inport
  Constant : Constant  Value=model.Parameters.NoiseGen.Modulator.FMA
  Constant1 : Constant  Value=model.Parameters.NoiseGen.Modulator.FMF
  Constant2 : Constant  Value=model.Parameters.NoiseGen.Modulator.FMPhi0
  Constant3 : Constant  Value=model.Parameters.NoiseGen.Modulator.FMK
  Digital Clock : DigitalClock  SampleTime=model.Parameters.NoiseGen.NoiseTs
  MATLAB Function : MATLAB Function  TreatAsAtomicUnit=on
  FM_Signal : Outport
  wires:
  Digital Clock/1 -> MATLAB Function/1(t)
  MATLAB Function/1(y) -> FM_Signal/1
  InputSignal/1 -> MATLAB Function/2(signal)
  Constant/1 -> MATLAB Function/3(A)
  Constant1/1 -> MATLAB Function/4(freq)
  Constant2/1 -> MATLAB Function/5(phi0)
  Constant3/1 -> MATLAB Function/6(K)

== system Simple_Model_Packaging_power_estimate/TransmissionChannel/NosieGen/调制方式/If Action Subsystem3 ==
  Jammer Source : Inport
  Action Port : ActionPort  ActionPortLabel=default:
  Out1 : Outport
  wires:
  Jammer Source/1 -> Out1/1

== system Simple_Model_Packaging_power_estimate/TransmissionChannel/NosieGen/调制方式/If Action Subsystem4 ==
  AM_Signal : Inport
  Action Port : ActionPort  ActionPortLabel=case [ 1 ]:
  Out1 : Outport
  wires:
  AM_Signal/1 -> Out1/1

== system Simple_Model_Packaging_power_estimate/TransmissionChannel/NosieGen/调制方式/If Action Subsystem5 ==
  PM_Signal : Inport
  Action Port : ActionPort  ActionPortLabel=case [ 2 ]:
  Out1 : Outport
  wires:
  PM_Signal/1 -> Out1/1

== system Simple_Model_Packaging_power_estimate/TransmissionChannel/NosieGen/调制方式/If Action Subsystem6 ==
  FM_Signal : Inport
  Action Port : ActionPort  ActionPortLabel=case [ 3 ]:
  Out1 : Outport
  wires:
  FM_Signal/1 -> Out1/1

== system Simple_Model_Packaging_power_estimate/TransmissionChannel/NosieGen/调制方式/PM ==
  InputSignal : Inport
  Constant : Constant  Value=model.Parameters.NoiseGen.Modulator.PMA
  Constant1 : Constant  Value=model.Parameters.NoiseGen.Modulator.PMF
  Constant2 : Constant  Value=model.Parameters.NoiseGen.Modulator.PMPhi0
  Constant3 : Constant  Value=model.Parameters.NoiseGen.Modulator.PMK
  Digital Clock : DigitalClock  SampleTime=model.Parameters.NoiseGen.NoiseTs
  MATLAB Function : MATLAB Function  TreatAsAtomicUnit=on
  PM_Signal : Outport
  wires:
  Digital Clock/1 -> MATLAB Function/1(t)
  InputSignal/1 -> MATLAB Function/2(signal)
  MATLAB Function/1(y) -> PM_Signal/1
  Constant/1 -> MATLAB Function/3(A)
  Constant1/1 -> MATLAB Function/4(freq)
  Constant3/1 -> MATLAB Function/5(K)
  Constant2/1 -> MATLAB Function/6(phi0)

== system Simple_Model_Packaging_power_estimate/TransmissionChannel/NosieGen/干扰方式/ChirpBasebandSignalGenerate/Frequency_Check ==
  ChirpSignal : Inport
  Derivative : Derivative
  Phase Extractor : dspsigops/Phase Extractor  TreatFramesIndependently=off  SimulateUsing=Code generation
  FrequencyConversionLine : Outport
  wires:
  ChirpSignal/1 -> Phase Extractor/1
  Phase Extractor/1 -> Derivative/1
  Derivative/1 -> FrequencyConversionLine/1

== matlab function Simple_Model_Packaging_power_estimate/TransmissionChannel/NosieGen/干扰源/PN MSK Noise/Random Binary Modulation ==
  data: cita_k input; MSKSignal output; t input; freq input
function MSKSignal = fcn(cita_k,t, freq)
    MSKSignal = cita_k * cos(2*pi*freq*t);
end

== matlab function Simple_Model_Packaging_power_estimate/TransmissionChannel/NosieGen/调制方式/PM/MATLAB Function ==
  data: t input; signal input; y output; A input; freq input; K input; phi0 input
function y = PM(t, signal, A, freq, K, phi0)
   y = A*cos(2*pi*freq*t+K*signal+phi0) ;
end

== matlab function Simple_Model_Packaging_power_estimate/TRsystem/跳频和频谱搬移/MATLAB Function ==
  data: y output; t input; fc input
function y = fcn(t,fc)
%     fs = 40e6;
%     Ts = 1/fs;
%     t = 0:Ts:0.002;
%     fc = 1e6;
    y = exp(1i*2*pi*fc*t);

end

== matlab function Simple_Model_Packaging_power_estimate/TransmissionChannel/NosieGen/干扰方式/ChirpBasebandSignalGenerate/Chirp_Signal_Generation ==
  data: y output; t input; f_chirp_min input; T_chirp input; k_chirp input
function y = ChirpSignal(t, f_chirp_min, T_chirp, k_chirp)
    t = mod(t,T_chirp);
    y = exp(1i*2*pi*(f_chirp_min*t+0.5*k_chirp*t^2));
end

== matlab function Simple_Model_Packaging_power_estimate/TransmissionChannel/NosieGen/干扰源/Monophonic Sine Noise/Monophonic_Generate ==
  data: t input; A input; freq input; monophonic output; phi0 input
function monophonic = MonophonicGenerate(t, A, freq, phi0)
    monophonic = A * sin(2*pi*freq*t+phi0);
end

== matlab function Simple_Model_Packaging_power_estimate/TransmissionChannel/NosieGen/调制方式/AM/AM_Carrier ==
  data: y output; t input; A input; freq input; phi0 input
function y = AM_Carrier(t, A, freq, phi0)
    y = A*cos(2*pi*freq*t+phi0);
end

== matlab function Simple_Model_Packaging_power_estimate/TransmissionChannel/NosieGen/调制方式/FM/MATLAB Function ==
  data: t input; signal input; y output; A input; freq input; phi0 input; K input
function y = FM(t, signal, A, freq, phi0, K)
   y = A*cos(2*pi*(freq+K*signal)*t+phi0) ;
end

== matlab function Simple_Model_Packaging_power_estimate/TransmissionChannel/NosieGen/干扰源/Random Binary Noise/Random Binary Modulation ==
  data: Jn input; Jt output; t input; A input; freq input; phi0 input
function Jt = fcn(Jn,t,A,freq,phi0)
    Jt = A*Jn*cos(2*pi*freq*t+phi0);
end

== matlab function Simple_Model_Packaging_power_estimate/TransmissionChannel/NosieGen/干扰源/Random Binary Noise/Unipolar to bipolar ==
  data: u input; Jn output
function Jn= fcn(u)
    Jn = 2*u-1;
end

== matlab function Simple_Model_Packaging_power_estimate/TransmissionChannel/NosieGen/干扰方式/StepSweepSignalGenerate/StepSweep_Signal ==
  data: y output; t input; f_stepSweep_min input; T_stepSweep input; delta_f_stepSweep input; T_stepSweep_dwell input; Ts input; N_stepSweep input
function y  = StepSweep(t, f_stepSweep_min, T_stepSweep, delta_f_stepSweep, T_stepSweep_dwell, Ts, N_stepSweep)
    a = mod(t,T_stepSweep)+Ts/10000;
    b = fix(a/T_stepSweep_dwell);
    if b == N_stepSweep
        b = N_stepSweep - 1;
    end
    f = (f_stepSweep_min+b*delta_f_stepSweep);
    y = exp(1i*2*pi*f*t);
end
